simulink model "TH4NIT2SOS"  (Simulink 10.0)
settings: Solver=ode45  StartTime=0.0  StopTime=40  FixedStep=0.01  RelTol=1e-5  EnableMultiTasking=on
libraries: truetime x4
settings Model: Creator=LIN  LastModifiedBy=peter
settings DataIOCC: LimitDataPoints=on
settings OptimizationCC: ExpressionDepthLimit=2147483647  InitFltsAndDblsToZero=on
settings DebuggingCC: SaveWithParameterizedLinksMsg=none  SignalResolutionControl=TryResolveAllWithWarning  SolverPrmCheckMsg=warning  MultiTaskDSMMsg=warning  MultiTaskCondExecSysMsg=none  StateNameClashWarn=warning
settings GRTTargetCC: TargetFcnLib=ansi_tfl_tmw.mat  GeneratePreprocessorConditionals=Disable all
settings ConfigComp: CovExternalEMLEnable=off

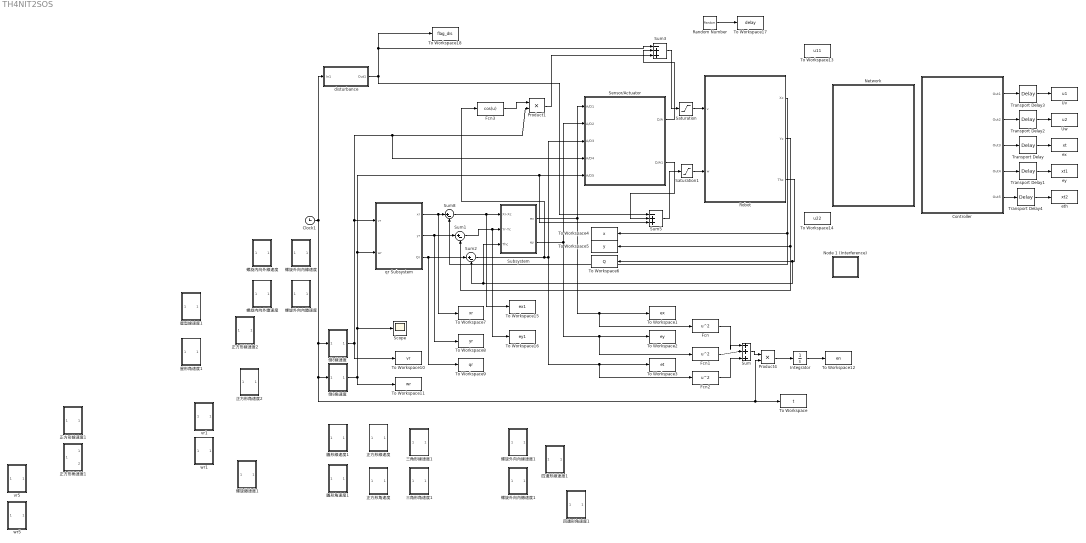
== system TH4NIT2SOS ==
  " Controller" : Subsystem
  " Sensor/Actuator" : Subsystem
  Clock1 : Clock
  Fcn : Fcn  Expr=u^2
  Fcn1 : Fcn  Expr=u^2
  Fcn2 : Fcn  Expr=u^2
  Fcn3 : Fcn  Expr=cos(u)
  Integrator : Integrator
  Network : Subsystem
  Node 1 (Interference) : Subsystem
  Product1 : Product  RndMeth=Zero
  Product4 : Product
  Random Number : RandomNumber  Variance=0.045  SampleTime=0.1
  Robot : Subsystem
  Saturation : Saturate  UpperLimit=1  LowerLimit=0
  Saturation1 : Saturate  UpperLimit=1.5  LowerLimit=-1.5
  Scope : Scope
  Subsystem : Subsystem
  Sum : Sum  Inputs=|+++
  Sum1 : Sum  Inputs=|+-
  Sum2 : Sum  Inputs=|+-
  Sum3 : Sum  Inputs=-++
  Sum5 : Sum  Inputs=-++
  Sum8 : Sum  Inputs=|+-
  To Workspace : ToWorkspace  VariableName=t  SampleTime=-1
  To Workspace1 : ToWorkspace  VariableName=ex  SampleTime=-1
  To Workspace10 : ToWorkspace  VariableName=vr  SampleTime=-1
  To Workspace11 : ToWorkspace  VariableName=wr  SampleTime=-1
  To Workspace12 : ToWorkspace  VariableName=en  SampleTime=-1
  To Workspace13 : ToWorkspace  VariableName=u11  SampleTime=-1
  To Workspace14 : ToWorkspace  VariableName=u22  SampleTime=-1
  To Workspace15 : ToWorkspace  VariableName=ex1  SampleTime=-1
  To Workspace16 : ToWorkspace  VariableName=ey1  SampleTime=-1
  To Workspace17 : ToWorkspace  VariableName=delay  SampleTime=-1
  To Workspace18 : ToWorkspace  VariableName=flag_dis  SampleTime=-1
  To Workspace2 : ToWorkspace  VariableName=ey  SampleTime=-1
  To Workspace3 : ToWorkspace  VariableName=et  SampleTime=-1
  To Workspace4 : ToWorkspace  VariableName=x  SampleTime=-1
  To Workspace5 : ToWorkspace  VariableName=y  SampleTime=-1
  To Workspace6 : ToWorkspace  VariableName=Q  SampleTime=-1
  To Workspace7 : ToWorkspace  VariableName=xr  SampleTime=-1
  To Workspace8 : ToWorkspace  VariableName=yr  SampleTime=-1
  To Workspace9 : ToWorkspace  VariableName=qr  SampleTime=-1
  Transport Delay{,1..4} (5 alike) : TransportDelay  BufferSize=5120
  Uv : ToWorkspace  VariableName=u1  SampleTime=-1
  Uw : ToWorkspace  VariableName=u2  SampleTime=-1
  disturbance : Subsystem
  eth : ToWorkspace  VariableName=xt2  SampleTime=-1
  ex : ToWorkspace  VariableName=xt  SampleTime=-1
  ey : ToWorkspace  VariableName=xt1  SampleTime=-1
  qr Subsystem : Subsystem
  vr1 : Subsystem
  vr5 : Subsystem
  wr1 : Subsystem
  wr5 : Subsystem
  三角形線速度1 : Subsystem
  三角形角速度1 : Subsystem
  倒8線速度 : Subsystem
  倒8角速度 : Subsystem
  四邊形線速度1 : Subsystem
  四邊形角速度1 : Subsystem
  圓形線速度1 : Subsystem
  圓形角速度1 : Subsystem
  星型線速度1 : Subsystem
  星形角速度1 : Subsystem
  正方形線速度 : Subsystem
  正方形線速度1 : Subsystem
  正方形線速度2 : Subsystem
  正方形角速度 : Subsystem
  正方形角速度1 : Subsystem
  正方形角速度2 : Subsystem
  螺旋內向外線速度 : Subsystem
  螺旋內向外繳速度 : Subsystem
  螺旋外向內線速度 : Subsystem
  螺旋外向內線速度1 : Subsystem
  螺旋外向內繳速度 : Subsystem
  螺旋外向內繳速度1 : Subsystem
  螺旋繳速度1 : Subsystem
  wires:
  倒8角速度/1(Out1) -> Scope/1, qr Subsystem/2(wr), Sum5/3, " Sensor/Actuator"/5(A/D5), To Workspace11/1
  " Controller"/3(Out3) -> Transport Delay/1
  " Controller"/2(Out2) -> Transport Delay2/1
  Robot/2(Yc) -> Sum1/2, To Workspace5/1
  disturbance/1(Out1) -> Sum5/1, To Workspace18/1, Sum3/1
  " Controller"/1(Out1) -> Transport Delay3/1
  Fcn1/1 -> Sum/2
  Sum/1 -> Product4/1
  Robot/3(Thc) -> Sum2/2, Subsystem/3(Thc), To Workspace6/1
  Sum1/1 -> To Workspace16/1, Subsystem/2(Yr-Yc)
  " Sensor/Actuator"/1(D/A) -> Sum3/2
  Sum2/1 -> " Sensor/Actuator"/3(A/D3), Fcn2/1, To Workspace3/1, Fcn3/1
  Product4/1 -> Integrator/1
  qr Subsystem/2(yr) -> Sum1/1, To Workspace8/1
  Sum8/1 -> To Workspace15/1, Subsystem/1(Xr-Xc)
  Clock1/1 -> 倒8線速度/1(In1), 倒8角速度/1(In1), Product4/2, To Workspace/1, disturbance/1(In1)
  Integrator/1 -> To Workspace12/1
  qr Subsystem/3(Qr) -> To Workspace9/1, Sum2/1
  Robot/1(Xc) -> Sum8/2, To Workspace4/1
  倒8線速度/1(Out1) -> To Workspace10/1, Product1/2, " Sensor/Actuator"/4(A/D4), qr Subsystem/1(vr)
  qr Subsystem/1(xr) -> Sum8/1, To Workspace7/1
  Subsystem/1(ex) -> " Sensor/Actuator"/1(A/D1), Fcn/1, To Workspace1/1
  Subsystem/2(ey) -> Fcn1/1, To Workspace2/1, " Sensor/Actuator"/2(A/D2)
  Fcn3/1 -> Product1/1
  Fcn/1 -> Sum/1
  Fcn2/1 -> Sum/3
  " Sensor/Actuator"/2(D/A1) -> Sum5/2
  Product1/1 -> Sum3/3
  Sum3/1 -> Saturation/1
  Sum5/1 -> Saturation1/1
  Random Number/1 -> To Workspace17/1
  Saturation/1 -> Robot/1(v)
  Saturation1/1 -> Robot/2(w)
  " Controller"/5(Out5) -> Transport Delay4/1
  Transport Delay4/1 -> eth/1
  Transport Delay1/1 -> ey/1
  " Controller"/4(Out4) -> Transport Delay1/1
  Transport Delay/1 -> ex/1
  Transport Delay2/1 -> Uw/1
  Transport Delay3/1 -> Uv/1

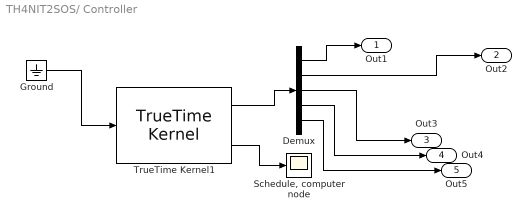
== system TH4NIT2SOS/ Controller ==
  Demux : Demux  Outputs=5
  Ground : Ground
  "Schedule, computer node" : Scope
  TrueTime Kernel1 : truetime/TrueTime Kernel  sfun=controllertest_init  args=[]  ninputsoutputs=[1 5]  ntriggers=0  trigtype=falling  nwnodenbr=3  clockoffsetdrift=[0 0]  schedoutput=on  battery=off  poweroutput=off  label=1: 3
  Out1 : Outport
  Out2 : Outport  Port=2
  Out3 : Outport  Port=3
  Out4 : Outport  Port=4
  Out5 : Outport  Port=5
  wires:
  TrueTime Kernel1/2 -> "Schedule, computer node"/1
  TrueTime Kernel1/1 -> Demux/1
  Demux/1 -> Out1/1
  Demux/2 -> Out2/1
  Ground/1 -> TrueTime Kernel1/1
  Demux/3 -> Out3/1
  Demux/4 -> Out4/1
  Demux/5 -> Out5/1

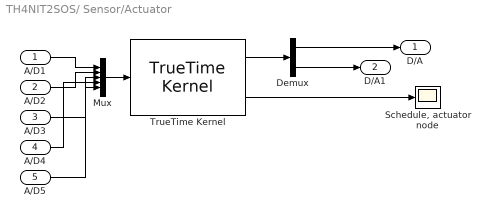
== system TH4NIT2SOS/ Sensor/Actuator ==
  A/D1 : Inport
  A/D2 : Inport  Port=2
  A/D3 : Inport  Port=3
  A/D4 : Inport  Port=4
  A/D5 : Inport  Port=5
  Demux : Demux  Outputs=2
  Mux : Mux  Inputs=5
  "Schedule, actuator node" : Scope
  TrueTime Kernel : truetime/TrueTime Kernel  sfun=actuator_init  args=[]  ninputsoutputs=[5 2]  ntriggers=0  trigtype=falling  nwnodenbr=2  clockoffsetdrift=[0 0]  schedoutput=on  battery=off  poweroutput=off  label=1: 2
  D/A : Outport
  D/A1 : Outport  Port=2
  wires:
  Demux/1 -> D/A/1
  TrueTime Kernel/1 -> Demux/1
  TrueTime Kernel/2 -> "Schedule, actuator node"/1
  A/D1/1 -> Mux/1
  A/D2/1 -> Mux/2
  A/D3/1 -> Mux/3
  Mux/1 -> TrueTime Kernel/1
  Demux/2 -> D/A1/1
  A/D4/1 -> Mux/4
  A/D5/1 -> Mux/5

== system TH4NIT2SOS/Network ==
  Network Schedule : Scope
  TrueTime Network : truetime/TrueTime Network  nwtype=CSMA/AMP (CAN)  nwnbr=1  nnodes=4  rate=80000  minsize=40  lossprob=0.5  seed=0  bandwidths=[1 0 0 0]  slotsize=20  schedule="[1 2 3  3 3 3]"  memsize=10000  buftype=Common buffer  overflow=Retransmit  dynSchedule=0  miniSlotSize=0  NIT=0  QSortMode=FIFO  sync=0  irtSchedule=0  nrtLength=0  nodeGraph=0  scheduleoutput=on
  wires:
  TrueTime Network/1 -> Network Schedule/1

== system TH4NIT2SOS/Node 1 (Interference) ==
  Ground1 : Ground
  "Schedule, interfering node" : Scope
  Terminator1 : Terminator
  TrueTime Kernel : truetime/TrueTime Kernel  sfun=interference_init  args=[]  ninputsoutputs=[1 1]  ntriggers=0  trigtype=falling  nwnodenbr=1  clockoffsetdrift=[0 0]  schedoutput=on  battery=off  poweroutput=off  label=1: 1
  wires:
  TrueTime Kernel/1 -> Terminator1/1
  TrueTime Kernel/2 -> "Schedule, interfering node"/1
  Ground1/1 -> TrueTime Kernel/1

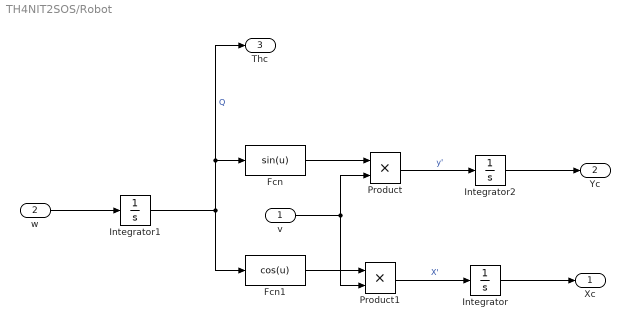
== system TH4NIT2SOS/Robot ==
  v : Inport
  w : Inport  Port=2
  Fcn : Fcn  Expr=sin(u)
  Fcn1 : Fcn  Expr=cos(u)
  Integrator : Integrator
  Integrator1 : Integrator  InitialCondition=0*pi/180
  Integrator2 : Integrator
  Product : Product  RndMeth=Zero
  Product1 : Product  RndMeth=Zero
  Xc : Outport
  Yc : Outport  Port=2
  Thc : Outport  Port=3
  wires:
  Fcn/1 -> Product/1
  Fcn1/1 -> Product1/1
  Integrator1/1 -> Fcn1/1, Fcn/1, Thc/1  "Q"
  Product/1 -> Integrator2/1  "y'"
  Product1/1 -> Integrator/1  "X'"
  v/1 -> Product/2, Product1/2
  w/1 -> Integrator1/1
  Integrator2/1 -> Yc/1
  Integrator/1 -> Xc/1

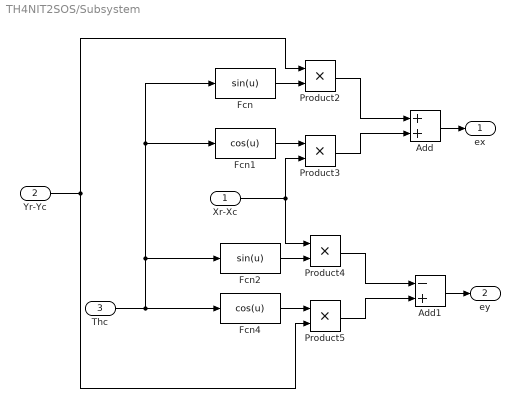
== system TH4NIT2SOS/Subsystem ==
  Xr-Xc : Inport
  Yr-Yc : Inport  Port=2
  Thc : Inport  Port=3
  Add : Sum
  Add1 : Sum  Inputs=-+
  Fcn : Fcn  Expr=sin(u)
  Fcn1 : Fcn  Expr=cos(u)
  Fcn2 : Fcn  Expr=sin(u)
  Fcn4 : Fcn  Expr=cos(u)
  Product{2..5} (4 alike) : Product  RndMeth=Zero
  ex : Outport
  ey : Outport  Port=2
  wires:
  Fcn/1 -> Product2/2
  Product2/1 -> Add/1
  Fcn1/1 -> Product3/1
  Product3/1 -> Add/2
  Fcn2/1 -> Product4/2
  Product4/1 -> Add1/1
  Fcn4/1 -> Product5/1
  Product5/1 -> Add1/2
  Add/1 -> ex/1
  Add1/1 -> ey/1
  Thc/1 -> Fcn4/1, Fcn1/1, Fcn/1, Fcn2/1
  Xr-Xc/1 -> Product3/2, Product4/1
  Yr-Yc/1 -> Product2/1, Product5/2

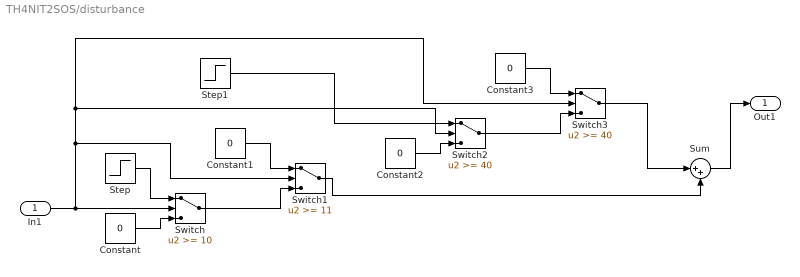
== system TH4NIT2SOS/disturbance ==
  In1 : Inport
  Constant{,1..3} (4 alike) : Constant  Value=0
  Step : Step  After=-0.8  SampleTime=0
  Step1 : Step  After=0.4  SampleTime=0
  Sum : Sum  Inputs=|++
  Switch : Switch  Threshold=10  ZeroCross=off
  Switch1 : Switch  Threshold=11
  Switch2 : Switch  Threshold=40  ZeroCross=off
  Switch3 : Switch  Threshold=40
  Out1 : Outport
  wires:
  Constant/1 -> Switch/3
  Switch/1 -> Switch1/3
  Constant1/1 -> Switch1/1
  Step/1 -> Switch/1
  In1/1 -> Switch3/2, Switch2/2, Switch1/2, Switch/2
  Constant2/1 -> Switch2/3
  Switch2/1 -> Switch3/3
  Constant3/1 -> Switch3/1
  Switch1/1 -> Sum/2
  Switch3/1 -> Sum/1
  Sum/1 -> Out1/1
  Step1/1 -> Switch2/1

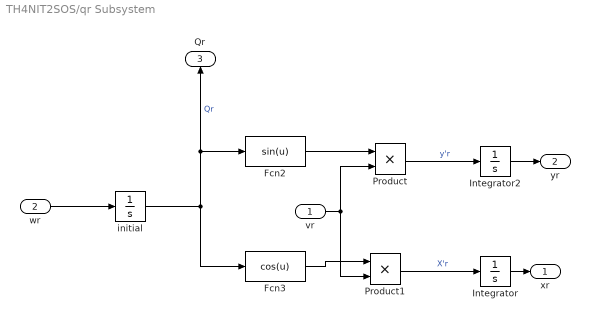
== system TH4NIT2SOS/qr Subsystem ==
  vr : Inport
  wr : Inport  Port=2
  Fcn2 : Fcn  Expr=sin(u)
  Fcn3 : Fcn  Expr=cos(u)
  Integrator : Integrator  InitialCondition=-0.5
  Integrator2 : Integrator  InitialCondition=-0.5
  Product : Product  RndMeth=Zero
  Product1 : Product  RndMeth=Zero
  initial : Integrator  InitialCondition=0*pi/180
  xr : Outport
  yr : Outport  Port=2
  Qr : Outport  Port=3
  wires:
  Fcn2/1 -> Product/1
  initial/1 -> Fcn3/1, Qr/1, Fcn2/1  "Qr"
  Product1/1 -> Integrator/1  "X'r"
  wr/1 -> initial/1
  Integrator2/1 -> yr/1
  Integrator/1 -> xr/1
  vr/1 -> Product/2, Product1/2
  Product/1 -> Integrator2/1  "y'r"
  Fcn3/1 -> Product1/1

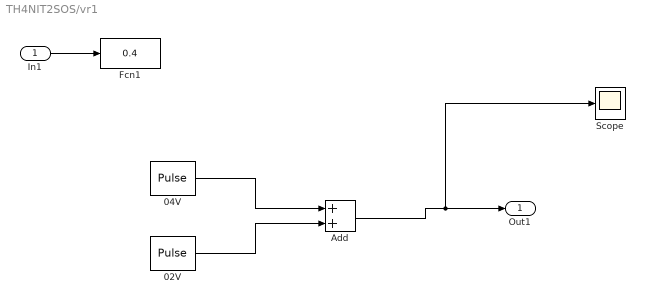
== system TH4NIT2SOS/vr1 ==
  In1 : Inport
  02V : DiscretePulseGenerator  PulseType=Time based  Amplitude=0.1  Period=12  PulseWidth=300/12  PhaseDelay=7
  04V : DiscretePulseGenerator  PulseType=Time based  Amplitude=0.4  Period=12  PulseWidth=900/12
  Add : Sum
  Fcn1 : Fcn  Expr=0.4
  Scope : Scope
  Out1 : Outport
  wires:
  In1/1 -> Fcn1/1
  04V/1 -> Add/1
  02V/1 -> Add/2
  Add/1 -> Scope/1, Out1/1

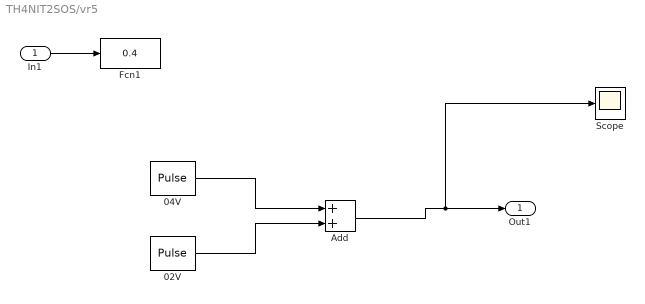
== system TH4NIT2SOS/vr5 ==
  In1 : Inport
  02V : DiscretePulseGenerator  PulseType=Time based  Amplitude=0  Period=12  PulseWidth=300/12
  04V : DiscretePulseGenerator  PulseType=Time based  Amplitude=0.4  Period=12  PulseWidth=900/12
  Add : Sum
  Fcn1 : Fcn  Expr=0.4
  Scope : Scope
  Out1 : Outport
  wires:
  In1/1 -> Fcn1/1
  04V/1 -> Add/1
  02V/1 -> Add/2
  Add/1 -> Scope/1, Out1/1

== system TH4NIT2SOS/wr1 ==
  In1 : Inport
  02V : DiscretePulseGenerator  PulseType=Time based  Amplitude=0.2  PulseWidth=50  PhaseDelay=1
  04V : DiscretePulseGenerator  PulseType=Time based  Amplitude=90*3.14159/180  Period=12  PulseWidth=300/12  PhaseDelay=7
  Fcn1 : Fcn  Expr=3*sin(0.05*u)
  Scope : Scope
  Out1 : Outport
  wires:
  In1/1 -> Fcn1/1
  04V/1 -> Scope/1, Out1/1

== system TH4NIT2SOS/wr5 ==
  In1 : Inport
  02V : DiscretePulseGenerator  PulseType=Time based  Amplitude=0.2  PulseWidth=50  PhaseDelay=1
  04V : DiscretePulseGenerator  PulseType=Time based  Amplitude=90*pi/180  Period=12  PulseWidth=300/12  PhaseDelay=9
  Fcn1 : Fcn  Expr=3*sin(0.05*u)
  Scope : Scope
  Out1 : Outport
  wires:
  In1/1 -> Fcn1/1
  04V/1 -> Scope/1, Out1/1

== system TH4NIT2SOS/三角形線速度1 ==
  In1 : Inport
  02V : DiscretePulseGenerator  PulseType=Time based  Amplitude=0  Period=12  PulseWidth=400/12
  04V : DiscretePulseGenerator  PulseType=Time based  Amplitude=0.4  Period=12  PulseWidth=800/12
  Add : Sum
  Scope : Scope
  Out1 : Outport
  wires:
  04V/1 -> Add/1
  02V/1 -> Add/2
  Add/1 -> Scope/1, Out1/1

== system TH4NIT2SOS/三角形角速度1 ==
  In1 : Inport
  04V : DiscretePulseGenerator  PulseType=Time based  Amplitude=120*pi/180  Period=12  PulseWidth=400/12  PhaseDelay=8
  Scope : Scope
  Out1 : Outport
  wires:
  04V/1 -> Scope/1, Out1/1

== system TH4NIT2SOS/倒8線速度 ==
  In1 : Inport
  Fcn1 : Fcn  Expr=0.5
  Out1 : Outport
  wires:
  Fcn1/1 -> Out1/1
  In1/1 -> Fcn1/1

== system TH4NIT2SOS/倒8角速度 ==
  In1 : Inport
  Fcn1 : Fcn  Expr=-sin(2*pi*u/15.118)
  Out1 : Outport
  wires:
  Fcn1/1 -> Out1/1
  In1/1 -> Fcn1/1

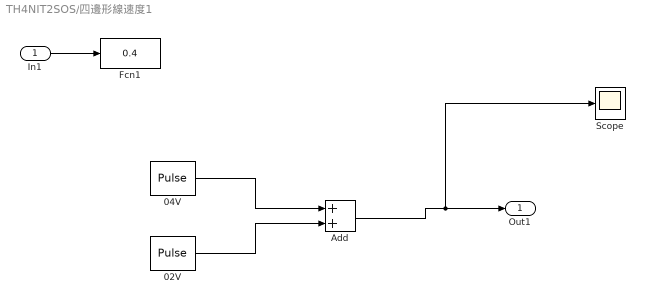
== system TH4NIT2SOS/四邊形線速度1 ==
  In1 : Inport
  02V : DiscretePulseGenerator  PulseType=Time based  Amplitude=0.1  Period=11  PulseWidth=300/11  PhaseDelay=7
  04V : DiscretePulseGenerator  PulseType=Time based  Amplitude=0.4  Period=11  PulseWidth=700/11
  Add : Sum
  Fcn1 : Fcn  Expr=0.4
  Scope : Scope
  Out1 : Outport
  wires:
  In1/1 -> Fcn1/1
  04V/1 -> Add/1
  02V/1 -> Add/2
  Add/1 -> Scope/1, Out1/1

== system TH4NIT2SOS/四邊形角速度1 ==
  In1 : Inport
  02V : DiscretePulseGenerator  PulseType=Time based  Amplitude=0.2  PulseWidth=50  PhaseDelay=1
  04V : DiscretePulseGenerator  PulseType=Time based  Amplitude=-30*3.14159/180  Period=11  PulseWidth=300/11  PhaseDelay=7
  Fcn1 : Fcn  Expr=3*sin(0.05*u)
  Scope : Scope
  Out1 : Outport
  wires:
  In1/1 -> Fcn1/1
  04V/1 -> Scope/1, Out1/1

== system TH4NIT2SOS/圓形線速度1 ==
  In1 : Inport
  Fcn1 : Fcn  Expr=0.5
  Out1 : Outport
  wires:
  Fcn1/1 -> Out1/1
  In1/1 -> Fcn1/1

== system TH4NIT2SOS/圓形角速度1 ==
  In1 : Inport
  Fcn1 : Fcn  Expr=0.5
  Out1 : Outport
  wires:
  Fcn1/1 -> Out1/1
  In1/1 -> Fcn1/1

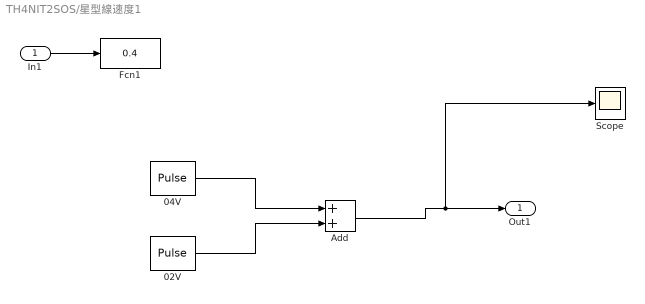
== system TH4NIT2SOS/星型線速度1 ==
  In1 : Inport
  02V : DiscretePulseGenerator  PulseType=Time based  Amplitude=0.1  Period=11  PulseWidth=300/11
  04V : DiscretePulseGenerator  PulseType=Time based  Amplitude=0.4  Period=11  PulseWidth=700/11
  Add : Sum
  Fcn1 : Fcn  Expr=0.4
  Scope : Scope
  Out1 : Outport
  wires:
  In1/1 -> Fcn1/1
  04V/1 -> Add/1
  02V/1 -> Add/2
  Add/1 -> Scope/1, Out1/1

== system TH4NIT2SOS/星形角速度1 ==
  In1 : Inport
  02V : DiscretePulseGenerator  PulseType=Time based  Amplitude=0.2  PulseWidth=50  PhaseDelay=1
  04V : DiscretePulseGenerator  PulseType=Time based  Amplitude=300*3.14159/180  Period=11  PulseWidth=288/11  PhaseDelay=7
  Fcn1 : Fcn  Expr=3*sin(0.05*u)
  Scope : Scope
  Out1 : Outport
  wires:
  In1/1 -> Fcn1/1
  04V/1 -> Scope/1, Out1/1

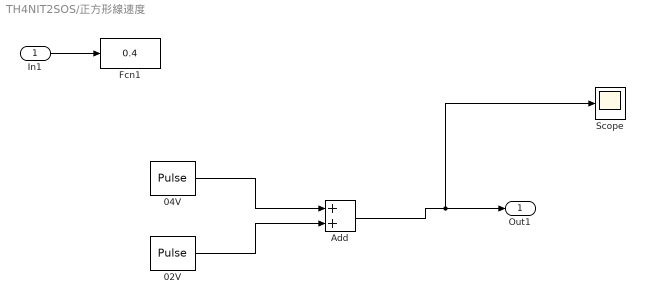
== system TH4NIT2SOS/正方形線速度 ==
  In1 : Inport
  02V : DiscretePulseGenerator  PulseType=Time based  Amplitude=0  Period=4  PulseWidth=25
  04V : DiscretePulseGenerator  PulseType=Time based  Amplitude=0.4  Period=4  PulseWidth=75
  Add : Sum
  Fcn1 : Fcn  Expr=0.4
  Scope : Scope
  Out1 : Outport
  wires:
  In1/1 -> Fcn1/1
  04V/1 -> Add/1
  02V/1 -> Add/2
  Add/1 -> Scope/1, Out1/1

== system TH4NIT2SOS/正方形線速度1 ==
  In1 : Inport
  02V : DiscretePulseGenerator  PulseType=Time based  Amplitude=0  Period=12  PulseWidth=300/12
  04V : DiscretePulseGenerator  PulseType=Time based  Amplitude=0.4  Period=12  PulseWidth=900/12
  Add : Sum
  Fcn1 : Fcn  Expr=0.4
  Scope : Scope
  Out1 : Outport
  wires:
  In1/1 -> Fcn1/1
  04V/1 -> Add/1
  02V/1 -> Add/2
  Add/1 -> Scope/1, Out1/1

== system TH4NIT2SOS/正方形線速度2 ==
  In1 : Inport
  02V : DiscretePulseGenerator  PulseType=Time based  Amplitude=0  Period=12  PulseWidth=300/12
  04V : DiscretePulseGenerator  PulseType=Time based  Amplitude=0.4  Period=12  PulseWidth=900/12
  Add : Sum
  Fcn1 : Fcn  Expr=0.4
  Scope : Scope
  Out1 : Outport
  wires:
  In1/1 -> Fcn1/1
  04V/1 -> Add/1
  02V/1 -> Add/2
  Add/1 -> Scope/1, Out1/1

== system TH4NIT2SOS/正方形角速度 ==
  In1 : Inport
  04V : DiscretePulseGenerator  PulseType=Time based  Amplitude=90*pi/180  Period=4  PulseWidth=25  PhaseDelay=3
  Scope : Scope
  Out1 : Outport
  wires:
  04V/1 -> Scope/1, Out1/1

== system TH4NIT2SOS/正方形角速度1 ==
  In1 : Inport
  02V : DiscretePulseGenerator  PulseType=Time based  Amplitude=0.2  PulseWidth=50  PhaseDelay=1
  04V : DiscretePulseGenerator  PulseType=Time based  Amplitude=90*pi/180  Period=12  PulseWidth=300/12  PhaseDelay=9
  Fcn1 : Fcn  Expr=3*sin(0.05*u)
  Scope : Scope
  Out1 : Outport
  Out2 : Outport  Port=2
  wires:
  In1/1 -> Fcn1/1
  04V/1 -> Scope/1, Out1/1

== system TH4NIT2SOS/正方形角速度2 ==
  In1 : Inport
  02V : DiscretePulseGenerator  PulseType=Time based  Amplitude=0.2  PulseWidth=50  PhaseDelay=1
  04V : DiscretePulseGenerator  PulseType=Time based  Amplitude=90*pi/180  Period=12  PulseWidth=300/12  PhaseDelay=9
  Fcn1 : Fcn  Expr=3*sin(0.05*u)
  Scope : Scope
  Out1 : Outport
  wires:
  In1/1 -> Fcn1/1
  04V/1 -> Scope/1, Out1/1

== system TH4NIT2SOS/螺旋內向外線速度 ==
  In1 : Inport
  Fcn1 : Fcn  Expr=0.5
  Out1 : Outport
  wires:
  Fcn1/1 -> Out1/1
  In1/1 -> Fcn1/1

== system TH4NIT2SOS/螺旋內向外繳速度 ==
  In1 : Inport
  Fcn1 : Fcn  Expr=1/(0.05*(u+10))
  Out1 : Outport
  wires:
  Fcn1/1 -> Out1/1
  In1/1 -> Fcn1/1

== system TH4NIT2SOS/螺旋外向內線速度 ==
  In1 : Inport
  Fcn1 : Fcn  Expr=0.5
  Out1 : Outport
  wires:
  Fcn1/1 -> Out1/1
  In1/1 -> Fcn1/1

== system TH4NIT2SOS/螺旋外向內線速度1 ==
  In1 : Inport
  Fcn1 : Fcn  Expr=0.3
  Out1 : Outport
  wires:
  Fcn1/1 -> Out1/1
  In1/1 -> Fcn1/1

== system TH4NIT2SOS/螺旋外向內繳速度 ==
  In1 : Inport
  Fcn1 : Fcn  Expr=0.015*u
  Out1 : Outport
  wires:
  Fcn1/1 -> Out1/1
  In1/1 -> Fcn1/1

== system TH4NIT2SOS/螺旋外向內繳速度1 ==
  In1 : Inport
  Fcn1 : Fcn  Expr=0.02*u
  Out1 : Outport
  wires:
  Fcn1/1 -> Out1/1
  In1/1 -> Fcn1/1

== system TH4NIT2SOS/螺旋繳速度1 ==
  In1 : Inport
  Fcn1 : Fcn  Expr=0.008*u
  Out1 : Outport
  wires:
  Fcn1/1 -> Out1/1
  In1/1 -> Fcn1/1
